simulink model "single_camera_xy_tracking_cv_ekf"  (R2025b)
settings: Solver=FixedStepDiscrete  StartTime=0  StopTime=T_end  FixedStep=Ts  RelTol=1e-3
InitFcn:
  | config_dir=fullfile(fileparts(get_param(bdroot,'FileName')),'..','config');
  | addpath(config_dir);
  | init_single_camera_xy_tracking_cv_ekf;
values from neighbouring files (symbols this model uses):
  Kpx = parameters(3)    [build_single_camera_joint_velocity_direct.m]    (also in build_single_camera_joint_velocity_direct1.m)
  Kpy = parameters(4);",  "k_ff=parameters(5)    [build_single_camera_joint_velocity_direct.m]    (also in build_single_camera_joint_velocity_direct1.m)
  Z_hat = parameters(2)    [build_single_camera_joint_velocity_direct.m]    (also in build_single_camera_joint_velocity_direct1.m)
undefined symbols (not defined in the file or in its folder): a_xy_max, command_velocity_timeout_sec, controller_enable, cx, cy, data, data_SL_Info, ekf_gate_threshold, ekf_reset_timeout_sec, enable_ekf_feedforward, enable_proportional, ff_ramp_time, fx, fy, joint_state_timeout_sec, k_ff, measurement_reset_timeout, P0, Q_ekf, R_ekf, required_valid_frames, target_timeout_sec, Ts, v_xy_max
libraries: ros2lib x5, robotmaniplib x3
Description:
  | Camera-frame 4-state CV Kalman Filter with commanded camera motion input.
settings Model: Creator=ASUS  LastModifiedBy=ASUS
settings DataIOCC: SignalLogging=off

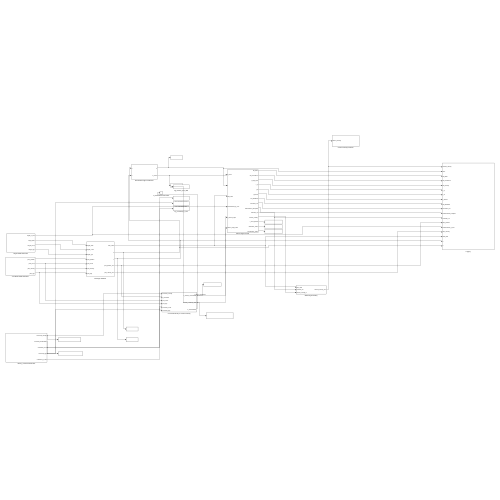
[thumbnail: Simulink's stored preview of the top-level diagram]
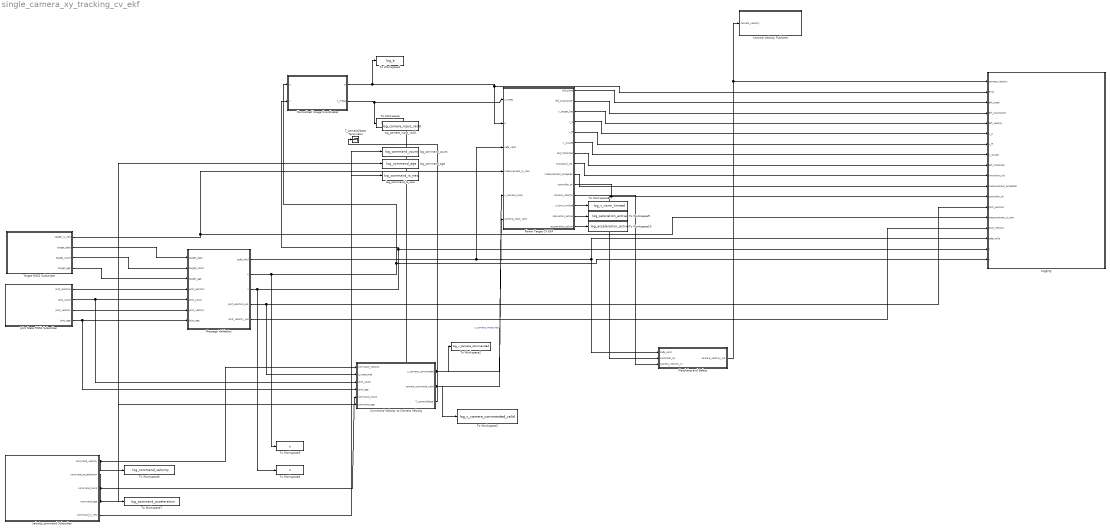
== system single_camera_xy_tracking_cv_ekf ==
  Camera Velocity Publisher : Subsystem
  Command Velocity to Camera Velocity : Subsystem
  Joint State ROS2 Subscriber : Subsystem
  Logging : Subsystem
  Message Validation : Subsystem
  Normalized Image Coordinates : Subsystem
  Planar Target CV EKF : Subsystem
  T_camera2base Terminator : Terminator
  Target ROS2 Subscriber : Subsystem
  To Workspace : ToWorkspace  VariableName=log_z_meas  SaveFormat=Timeseries  SampleTime=-1
  To Workspace1 : ToWorkspace  VariableName=log_e  SaveFormat=Timeseries  SampleTime=-1
  To Workspace10 : ToWorkspace  VariableName=log_acceleration_active  SaveFormat=Timeseries  SampleTime=-1
  To Workspace2 : ToWorkspace  VariableName=log_v_camera_commanded  SaveFormat=Timeseries  SampleTime=-1
  To Workspace3 : ToWorkspace  VariableName=log_v_camera_commanded_valid  SaveFormat=Timeseries  SampleTime=-1
  To Workspace4 : ToWorkspace  VariableName=v  SaveFormat=Timeseries  SampleTime=-1
  To Workspace5 : ToWorkspace  VariableName=u  SaveFormat=Timeseries  SampleTime=-1
  To Workspace6 : ToWorkspace  VariableName=log_command_velocity  SaveFormat=Timeseries  SampleTime=-1
  To Workspace7 : ToWorkspace  VariableName=log_command_acceleration  SaveFormat=Timeseries  SampleTime=-1
  To Workspace8 : ToWorkspace  VariableName=log_v_norm_limited  SaveFormat=Timeseries  SampleTime=-1
  To Workspace9 : ToWorkspace  VariableName=log_saturation_active  SaveFormat=Timeseries  SampleTime=-1
  Watchdog and Safety : Subsystem
  log_camera_input_valid : ToWorkspace  VariableName=log_camera_input_valid  SaveFormat=Timeseries  SampleTime=-1
  log_command_age : ToWorkspace  VariableName=log_command_age  SaveFormat=Timeseries  SampleTime=-1
  log_command_count : ToWorkspace  VariableName=log_command_count  SaveFormat=Timeseries  SampleTime=-1
  log_command_is_new : ToWorkspace  VariableName=log_command_is_new  SaveFormat=Timeseries  SampleTime=-1
  velocity_command Subscriber : Subsystem
  wires:
  Target ROS2 Subscriber/4(target_age) -> Message Validation/3(target_age)
  Target ROS2 Subscriber/2(target_data) -> Message Validation/1(target_data)
  Target ROS2 Subscriber/3(target_count) -> Message Validation/2(target_count)
  Planar Target CV EKF/3(v_target_hat) -> Logging/5(ekf_velocity)
  Message Validation/2(u) -> Normalized Image Coordinates/1(u), Logging/18(u), To Workspace5/1
  Planar Target CV EKF/10(controller_ok) -> Watchdog and Safety/2(controller_ok), Logging/12(controller_ok)
  Joint State ROS2 Subscriber/4(joint_age) -> Command Velocity to Camera Velocity/4(joint_age), Message Validation/7(joint_age)
  Joint State ROS2 Subscriber/2(joint_count) -> Command Velocity to Camera Velocity/3(joint_count), Message Validation/5(joint_count)
  Joint State ROS2 Subscriber/1(joint_position) -> Message Validation/4(joint_position)
  Joint State ROS2 Subscriber/3(joint_velocity) -> Message Validation/6(joint_velocity)
  Message Validation/1(safe_valid) -> Logging/16(safe_valid), Watchdog and Safety/1(safe_valid), Planar Target CV EKF/3(safe_valid)
  Message Validation/3(v) -> To Workspace4/1, Normalized Image Coordinates/2(v), Logging/17(v)
  Message Validation/4(joint_position_out) -> Command Velocity to Camera Velocity/2(q_measured), Logging/13(joint_position)
  Message Validation/5(joint_velocity_out) -> Logging/15(joint_velocity)
  Normalized Image Coordinates/1(e) -> To Workspace1/1, Logging/2(error), Planar Target CV EKF/2(e)
  Normalized Image Coordinates/2(z_meas) -> To Workspace/1, Planar Target CV EKF/1(z_meas)
  Planar Target CV EKF/1(ekf_state) -> Logging/3(ekf_state)
  Planar Target CV EKF/2(ekf_covariance) -> Logging/4(ekf_covariance)
  Planar Target CV EKF/9(measurement_accepted) -> Logging/11(measurement_accepted)
  Planar Target CV EKF/7(ekf_initialized) -> Logging/9(ekf_initialized)
  Planar Target CV EKF/8(innovation_nis) -> Logging/10(innovation_nis)
  Planar Target CV EKF/4(v_p) -> Logging/6(v_p)
  Planar Target CV EKF/5(v_ff) -> Logging/7(v_ff)
  Planar Target CV EKF/6(v_issued) -> Logging/8(v_issued)
  Planar Target CV EKF/11(camera_velocity) -> Watchdog and Safety/3(camera_velocity_in)
  Watchdog and Safety/1(camera_velocity_out) -> Camera Velocity Publisher/1(camera_velocity), Logging/1(camera_velocity)
  Target ROS2 Subscriber/1(target_is_new) -> Planar Target CV EKF/4(measurement_is_new), Logging/14(measurement_is_new)
  Command Velocity to Camera Velocity/1(v_camera_commanded) -> To Workspace2/1, Planar Target CV EKF/5(v_camera_input)  "v_camera_measured"
  Command Velocity to Camera Velocity/2(camera_command_valid) -> To Workspace3/1, Planar Target CV EKF/6(camera_input_valid), log_camera_input_valid/1
  velocity_command Subscriber/1(command_velocity) -> To Workspace6/1, Command Velocity to Camera Velocity/1(command_velocity)
  velocity_command Subscriber/2(command_acceleration) -> To Workspace7/1
  Planar Target CV EKF/12(v_norm_limited) -> To Workspace8/1
  Planar Target CV EKF/13(saturation_active) -> To Workspace9/1
  Planar Target CV EKF/14(acceleration_active) -> To Workspace10/1
  velocity_command Subscriber/3(command_count) -> Command Velocity to Camera Velocity/5(command_count), log_command_count/1
  velocity_command Subscriber/4(command_age) -> Command Velocity to Camera Velocity/6(command_age), log_command_age/1
  Command Velocity to Camera Velocity/3(T_camera2base) -> T_camera2base Terminator/1
  velocity_command Subscriber/5(command_is_new) -> log_command_is_new/1

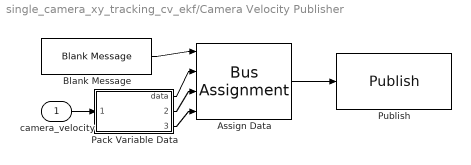
== system single_camera_xy_tracking_cv_ekf/Camera Velocity Publisher ==
  camera_velocity : Inport
  Assign Data : BusAssignment  AssignedSignals=data,data_SL_Info.CurrentLength,data_SL_Info.ReceivedLength
  Blank Message : ros2lib/Blank Message  messageClass=Message  entityType=std_msgs/Float64MultiArray  messageType=std_msgs/Float64MultiArray  SampleTime=Ts
  Pack Variable Data : MATLAB Function  TreatAsAtomicUnit=on
  Publish : ros2lib/Publish  topicSource=Select from ROS network  topic=/simulink/camera_velocity  messageType=std_msgs/Float64MultiArray  QOSHistory=Keep last  QOSDepth=1  QOSReliability=Reliable  QOSDurability=Volatile  QOSDeadline=Inf  QOSLifespan=Inf  QOSLiveliness=Automatic  QOSLeaseDuration=Inf  QOSAvoidROSNamespaceConventions=off
  wires:
  Blank Message/1 -> Assign Data/1
  Assign Data/1 -> Publish/1
  camera_velocity/1 -> Pack Variable Data/1(camera_velocity)
  Pack Variable Data/1(data) -> Assign Data/2
  Pack Variable Data/2(current_length) -> Assign Data/3
  Pack Variable Data/3(received_length) -> Assign Data/4

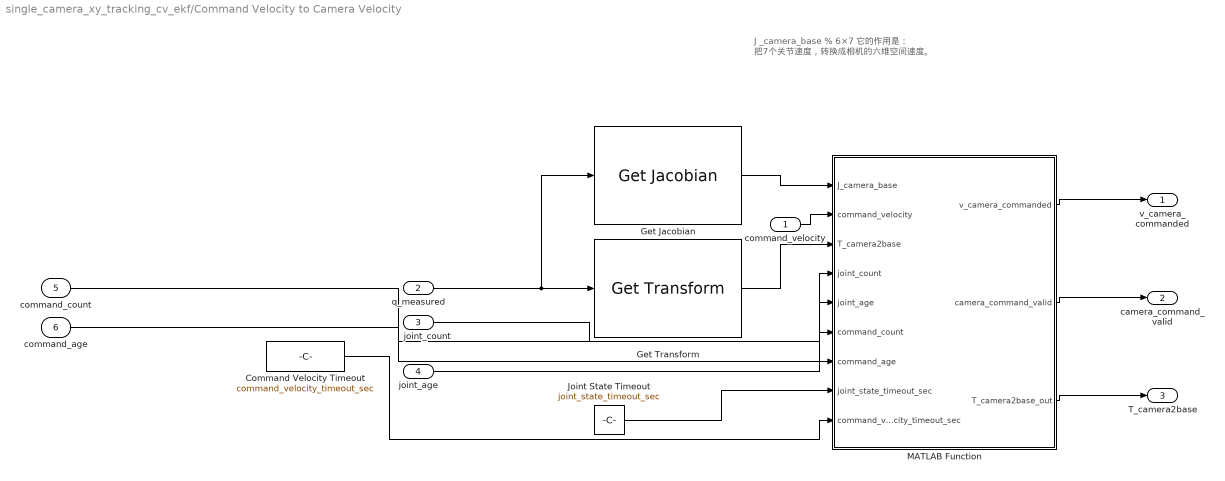
== system single_camera_xy_tracking_cv_ekf/Command Velocity to Camera Velocity ==
  note: J _camera_base % 6×7
      | 它的作用是：
      | 把7个关节速度，转换成相机的六维空间速度。
  command_velocity : Inport
  q_measured : Inport  Port=2
  joint_count : Inport  Port=3
  joint_age : Inport  Port=4
  command_count : Inport  Port=5
  command_age : Inport  Port=6
  Command Velocity Timeout : Constant  Value=command_velocity_timeout_sec
  Get Jacobian : robotmaniplib/Get Jacobian  RigidBodyTree=fr3_camera_robot  EndEffector=camera_link  SimulateUsing=Interpreted execution
  Get Transform : robotmaniplib/Get Transform  RigidBodyTree=fr3_camera_robot  SourceBody=camera_link  TargetBody=base  SimulateUsing=Interpreted execution
  Joint State Timeout : Constant  Value=joint_state_timeout_sec
  MATLAB Function : MATLAB Function  TreatAsAtomicUnit=on
  v_camera_commanded : Outport
  camera_command_valid : Outport  Port=2
  T_camera2base : Outport  Port=3
  wires:
  q_measured/1 -> Get Jacobian/1, Get Transform/1
  MATLAB Function/1(v_camera_commanded) -> v_camera_commanded/1
  MATLAB Function/2(camera_command_valid) -> camera_command_valid/1
  MATLAB Function/3(T_camera2base_out) -> T_camera2base/1
  Get Jacobian/1 -> MATLAB Function/1(J_camera_base)
  command_velocity/1 -> MATLAB Function/2(command_velocity)
  Get Transform/1 -> MATLAB Function/3(T_camera2base)
  joint_count/1 -> MATLAB Function/4(joint_count)
  joint_age/1 -> MATLAB Function/5(joint_age)
  command_count/1 -> MATLAB Function/6(command_count)
  command_age/1 -> MATLAB Function/7(command_age)
  Joint State Timeout/1 -> MATLAB Function/8(joint_state_timeout_sec)
  Command Velocity Timeout/1 -> MATLAB Function/9(command_velocity_timeout_sec)

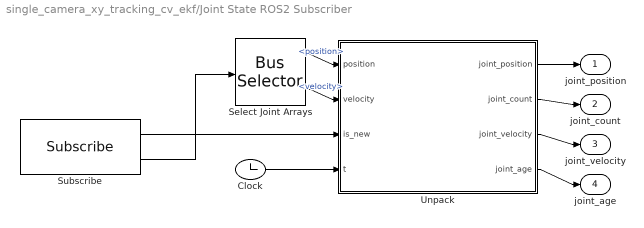
== system single_camera_xy_tracking_cv_ekf/Joint State ROS2 Subscriber ==
  Clock : Clock
  Select Joint Arrays : BusSelector  OutputSignals=position,velocity
  Subscribe : ros2lib/Subscribe  topicSource=Select from ROS network  topic=/franka/joint_states  messageType=sensor_msgs/JointState  sampleTime=Ts  QOSHistory=Keep last  QOSDepth=1  QOSReliability=Best effort  QOSDurability=Volatile  QOSDeadline=Inf  QOSLifespan=Inf  QOSLiveliness=Automatic  QOSLeaseDuration=Inf  QOSAvoidROSNamespaceConventions=off
  Unpack : MATLAB Function  TreatAsAtomicUnit=on
  joint_position : Outport
  joint_count : Outport  Port=2
  joint_velocity : Outport  Port=3
  joint_age : Outport  Port=4
  wires:
  Unpack/1(joint_position) -> joint_position/1
  Unpack/2(joint_count) -> joint_count/1
  Unpack/3(joint_velocity) -> joint_velocity/1
  Unpack/4(joint_age) -> joint_age/1
  Select Joint Arrays/1 -> Unpack/1(position)  "<position>"
  Select Joint Arrays/2 -> Unpack/2(velocity)  "<velocity>"
  Clock/1 -> Unpack/4(t)
  Subscribe/2 -> Select Joint Arrays/1
  Subscribe/1 -> Unpack/3(is_new)

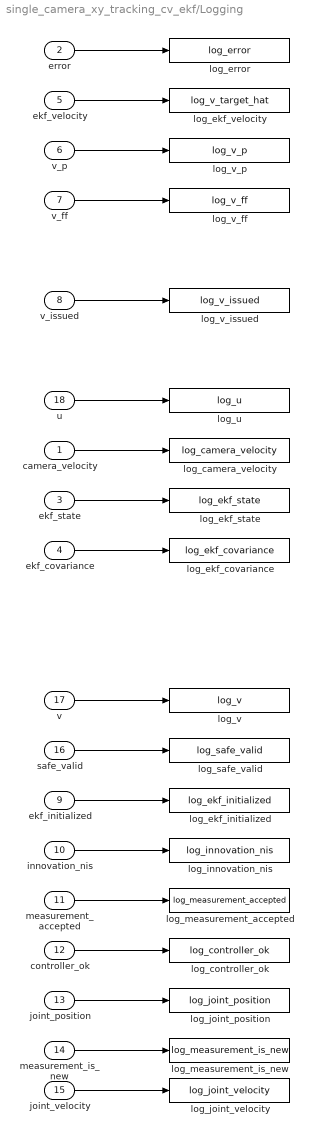
== system single_camera_xy_tracking_cv_ekf/Logging ==
  camera_velocity : Inport
  error : Inport  Port=2
  ekf_state : Inport  Port=3
  ekf_covariance : Inport  Port=4
  ekf_velocity : Inport  Port=5
  v_p : Inport  Port=6
  v_ff : Inport  Port=7
  v_issued : Inport  Port=8
  ekf_initialized : Inport  Port=9
  innovation_nis : Inport  Port=10
  measurement_accepted : Inport  Port=11
  controller_ok : Inport  Port=12
  joint_position : Inport  Port=13
  measurement_is_new : Inport  Port=14
  joint_velocity : Inport  Port=15
  safe_valid : Inport  Port=16
  v : Inport  Port=17
  u : Inport  Port=18
  log_camera_velocity : ToWorkspace  VariableName=log_camera_velocity  SaveFormat=Structure With Time  SampleTime=-1
  log_controller_ok : ToWorkspace  VariableName=log_controller_ok  SaveFormat=Structure With Time  SampleTime=-1
  log_ekf_covariance : ToWorkspace  VariableName=log_ekf_covariance  SaveFormat=Structure With Time  SampleTime=-1
  log_ekf_initialized : ToWorkspace  VariableName=log_ekf_initialized  SaveFormat=Structure With Time  SampleTime=-1
  log_ekf_state : ToWorkspace  VariableName=log_ekf_state  SaveFormat=Structure With Time  SampleTime=-1
  log_ekf_velocity : ToWorkspace  VariableName=log_v_target_hat  SaveFormat=Structure With Time  SampleTime=-1
  log_error : ToWorkspace  VariableName=log_error  SaveFormat=Structure With Time  SampleTime=-1
  log_innovation_nis : ToWorkspace  VariableName=log_innovation_nis  SaveFormat=Structure With Time  SampleTime=-1
  log_joint_position : ToWorkspace  VariableName=log_joint_position  SaveFormat=Structure With Time  SampleTime=-1
  log_joint_velocity : ToWorkspace  VariableName=log_joint_velocity  SaveFormat=Structure With Time  SampleTime=-1
  log_measurement_accepted : ToWorkspace  VariableName=log_measurement_accepted  SaveFormat=Structure With Time  SampleTime=-1
  log_measurement_is_new : ToWorkspace  VariableName=log_measurement_is_new  SaveFormat=Structure With Time  SampleTime=-1
  log_safe_valid : ToWorkspace  VariableName=log_safe_valid  SaveFormat=Structure With Time  SampleTime=-1
  log_u : ToWorkspace  VariableName=log_u  SaveFormat=Structure With Time  SampleTime=-1
  log_v : ToWorkspace  VariableName=log_v  SaveFormat=Structure With Time  SampleTime=-1
  log_v_ff : ToWorkspace  VariableName=log_v_ff  SaveFormat=Structure With Time  SampleTime=-1
  log_v_issued : ToWorkspace  VariableName=log_v_issued  SaveFormat=Structure With Time  SampleTime=-1
  log_v_p : ToWorkspace  VariableName=log_v_p  SaveFormat=Structure With Time  SampleTime=-1
  wires:
  error/1 -> log_error/1
  ekf_velocity/1 -> log_ekf_velocity/1
  v_p/1 -> log_v_p/1
  v_ff/1 -> log_v_ff/1
  v_issued/1 -> log_v_issued/1
  u/1 -> log_u/1
  camera_velocity/1 -> log_camera_velocity/1
  ekf_state/1 -> log_ekf_state/1
  ekf_covariance/1 -> log_ekf_covariance/1
  v/1 -> log_v/1
  safe_valid/1 -> log_safe_valid/1
  ekf_initialized/1 -> log_ekf_initialized/1
  innovation_nis/1 -> log_innovation_nis/1
  measurement_accepted/1 -> log_measurement_accepted/1
  controller_ok/1 -> log_controller_ok/1
  joint_position/1 -> log_joint_position/1
  joint_velocity/1 -> log_joint_velocity/1
  measurement_is_new/1 -> log_measurement_is_new/1

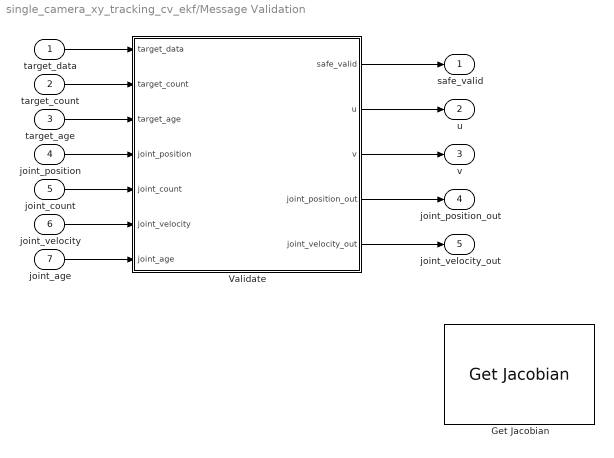
== system single_camera_xy_tracking_cv_ekf/Message Validation ==
  target_data : Inport
  target_count : Inport  Port=2
  target_age : Inport  Port=3
  joint_position : Inport  Port=4
  joint_count : Inport  Port=5
  joint_velocity : Inport  Port=6
  joint_age : Inport  Port=7
  Get Jacobian : robotmaniplib/Get Jacobian  RigidBodyTree=twoJointRigidBodyTree  EndEffector=tool  SimulateUsing=Interpreted execution
  Validate : MATLAB Function  TreatAsAtomicUnit=on
  safe_valid : Outport
  u : Outport  Port=2
  v : Outport  Port=3
  joint_position_out : Outport  Port=4
  joint_velocity_out : Outport  Port=5
  wires:
  Validate/1(safe_valid) -> safe_valid/1
  Validate/2(u) -> u/1
  Validate/3(v) -> v/1
  Validate/4(joint_position_out) -> joint_position_out/1
  Validate/5(joint_velocity_out) -> joint_velocity_out/1
  target_data/1 -> Validate/1(target_data)
  target_count/1 -> Validate/2(target_count)
  target_age/1 -> Validate/3(target_age)
  joint_position/1 -> Validate/4(joint_position)
  joint_count/1 -> Validate/5(joint_count)
  joint_velocity/1 -> Validate/6(joint_velocity)
  joint_age/1 -> Validate/7(joint_age)

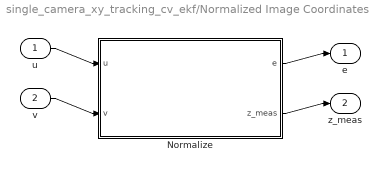
== system single_camera_xy_tracking_cv_ekf/Normalized Image Coordinates ==
  u : Inport
  v : Inport  Port=2
  Normalize : MATLAB Function  TreatAsAtomicUnit=on
  e : Outport
  z_meas : Outport  Port=2
  wires:
  u/1 -> Normalize/1(u)
  v/1 -> Normalize/2(v)
  Normalize/1(e) -> e/1
  Normalize/2(z_meas) -> z_meas/1

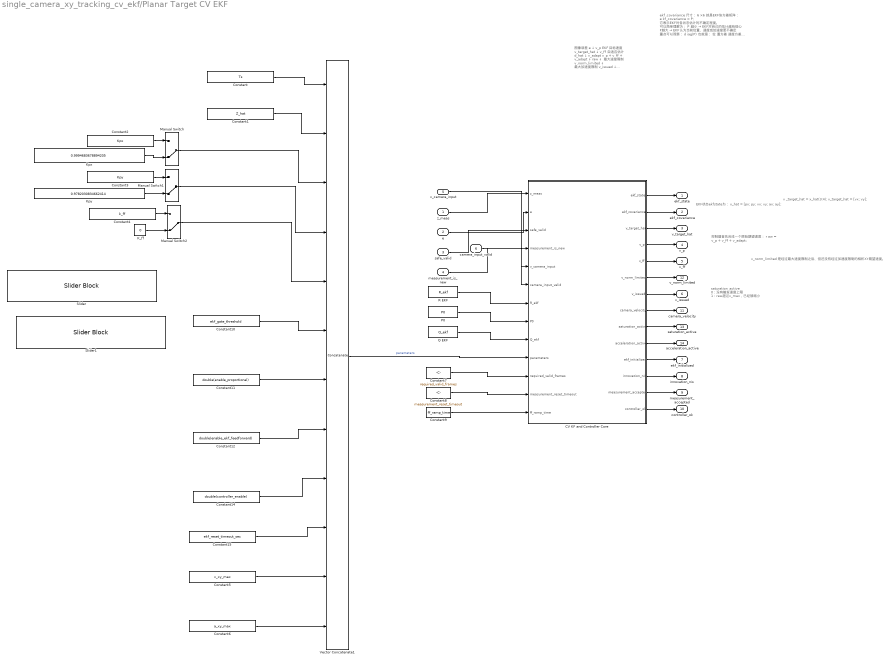
== system single_camera_xy_tracking_cv_ekf/Planar Target CV EKF ==
  note: saturation_active
      | 0：没有触发速度上限
      | 1：raw超过v_max，已经被缩小
  note: ekf_covariance
      | 尺寸：
      | 6 ×6
      | 就是EKF协方差矩阵：
      | e kf_covariance = P;
      | 它表示EKF对各状态估计的不确定程度。
      | 可以简单理解为：
      | P 越小
      | → EKF对自己的估计越有信心
      |
      | P越大
      | → EKF认为当前位置、速度或加速度更不确定
      | 重点可以观察：
      | d iag(P)
      | 也就是：
      | 位 置方差
      | 速度方差
      | 加速度方差
  note: 图像误差 e
      |     ↓
      | v_p
      |
      | EKF目标速度 v_target_hat
      |     ↓
      | v_ff
      |
      | 自适应估计 d_hat
      |     ↓
      | v_adapt
      |
      | v_p + v_ff + v_adapt
      |     ↓
      | raw
      |     ↓ 最大速度限制
      | v_norm_limited
      |     ↓ 最大加速度限制
      | v_issued
      |     ↓ 扩展为6维
      | camera_velocity
  note: EKF状态ekfstate为： x_hat = [px; py; vx; vy; ax; ay];
  note: v _target_hat = x_hat(3:4); v_target_hat = [vx; vy];
  note: 控制器首先合成一个原始期望速度：
      | r aw = v_p + v_ff + v_adapt;
  note: v_norm_limited 是经过最大速度限制之后、但还没有经过加速度限制的相机XY期望速度。
  z_meas : Inport
  e : Inport  Port=2
  safe_valid : Inport  Port=3
  measurement_is_new : Inport  Port=4
  v_camera_input : Inport  Port=5
  camera_input_valid : Inport  Port=6
  CV KF and Controller Core : MATLAB Function  TreatAsAtomicUnit=on
  Constant : Constant  Value=Ts
  Constant1 : Constant  Value=Z_hat
  Constant10 : Constant  Value=ekf_gate_threshold
  Constant11 : Constant  Value=double(enable_proportional)
  Constant12 : Constant  Value=double(enable_ekf_feedforward)
  Constant14 : Constant  Value=double(controller_enable)
  Constant15 : Constant  Value=ekf_reset_timeout_sec
  Constant2 : Constant  Value=Kpx
  Constant3 : Constant  Value=Kpy
  Constant4 : Constant  Value=k_ff
  Constant5 : Constant  Value=v_xy_max
  Constant6 : Constant  Value=a_xy_max
  Constant7 : Constant  Value=required_valid_frames
  Constant8 : Constant  Value=measurement_reset_timeout
  Constant9 : Constant  Value=ff_ramp_time
  K_ff : Constant  Value=0
  Kpx : Constant  Value=0.9994683678894205
  Kpy : Constant  Value=0.9782030834662414
  Manual Switch : ManualSwitch  CurrentSetting=0
  Manual Switch1 : ManualSwitch  CurrentSetting=0
  Manual Switch2 : ManualSwitch  CurrentSetting=0
  P0 : Constant  Value=P0
  Q EKF : Constant  Value=Q_ekf
  R EKF : Constant  Value=R_ekf
  Slider : SliderBlock  ScaleMax=10
  Slider1 : SliderBlock  ScaleMax=10
  Vector Concatenate1 : Concatenate  NumInputs=12
  ekf_state : Outport
  ekf_covariance : Outport  Port=2
  v_target_hat : Outport  Port=3
  v_p : Outport  Port=4
  v_ff : Outport  Port=5
  v_issued : Outport  Port=6
  ekf_initialized : Outport  Port=7
  innovation_nis : Outport  Port=8
  measurement_accepted : Outport  Port=9
  controller_ok : Outport  Port=10
  camera_velocity : Outport  Port=11
  v_norm_limited : Outport  Port=12
  saturation_active : Outport  Port=13
  acceleration_active : Outport  Port=14
  wires:
  CV KF and Controller Core/1(ekf_state) -> ekf_state/1
  CV KF and Controller Core/2(ekf_covariance) -> ekf_covariance/1
  CV KF and Controller Core/3(v_target_hat) -> v_target_hat/1
  CV KF and Controller Core/4(v_p) -> v_p/1
  CV KF and Controller Core/5(v_ff) -> v_ff/1
  CV KF and Controller Core/7(v_issued) -> v_issued/1
  CV KF and Controller Core/8(camera_velocity) -> camera_velocity/1
  CV KF and Controller Core/11(ekf_initialized) -> ekf_initialized/1
  CV KF and Controller Core/12(innovation_nis) -> innovation_nis/1
  CV KF and Controller Core/13(measurement_accepted) -> measurement_accepted/1
  CV KF and Controller Core/14(controller_ok) -> controller_ok/1
  Constant/1 -> Vector Concatenate1/1
  Constant1/1 -> Vector Concatenate1/2
  Constant10/1 -> Vector Concatenate1/6
  Constant11/1 -> Vector Concatenate1/7
  Constant12/1 -> Vector Concatenate1/8
  Constant14/1 -> Vector Concatenate1/9
  Constant15/1 -> Vector Concatenate1/10
  Constant2/1 -> Manual Switch/1
  Manual Switch/1 -> Vector Concatenate1/3
  Kpx/1 -> Manual Switch/2
  Kpy/1 -> Manual Switch1/2
  Constant3/1 -> Manual Switch1/1
  Manual Switch1/1 -> Vector Concatenate1/4
  Constant4/1 -> Manual Switch2/1
  Manual Switch2/1 -> Vector Concatenate1/5
  K_ff/1 -> Manual Switch2/2
  CV KF and Controller Core/6(v_norm_limited) -> v_norm_limited/1
  CV KF and Controller Core/10(acceleration_active) -> acceleration_active/1
  CV KF and Controller Core/9(saturation_active) -> saturation_active/1
  Constant6/1 -> Vector Concatenate1/12
  Constant5/1 -> Vector Concatenate1/11
  z_meas/1 -> CV KF and Controller Core/1(z_meas)
  e/1 -> CV KF and Controller Core/2(e)
  safe_valid/1 -> CV KF and Controller Core/3(safe_valid)
  measurement_is_new/1 -> CV KF and Controller Core/4(measurement_is_new)
  v_camera_input/1 -> CV KF and Controller Core/5(v_camera_input)
  camera_input_valid/1 -> CV KF and Controller Core/6(camera_input_valid)
  R EKF/1 -> CV KF and Controller Core/7(R_ekf)
  P0/1 -> CV KF and Controller Core/8(P0)
  Q EKF/1 -> CV KF and Controller Core/9(Q_ekf)
  Vector Concatenate1/1 -> CV KF and Controller Core/10(parameters)  "parameters"
  Constant7/1 -> CV KF and Controller Core/11(required_valid_frames)
  Constant8/1 -> CV KF and Controller Core/12(measurement_reset_timeout)
  Constant9/1 -> CV KF and Controller Core/13(ff_ramp_time)

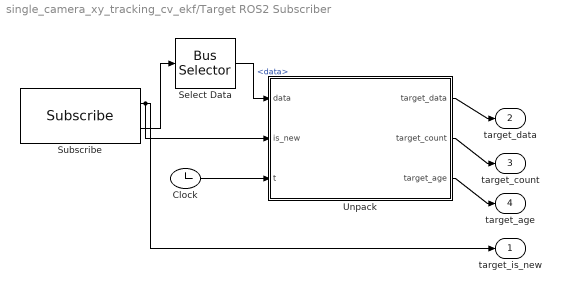
== system single_camera_xy_tracking_cv_ekf/Target ROS2 Subscriber ==
  Clock : Clock
  Select Data : BusSelector  OutputSignals=data
  Subscribe : ros2lib/Subscribe  topicSource=Select from ROS network  topic=/apriltag_detector/target_position  messageType=std_msgs/Float64MultiArray  sampleTime=Ts  QOSHistory=Keep last  QOSDepth=1  QOSReliability=Best effort  QOSDurability=Volatile  QOSDeadline=Inf  QOSLifespan=Inf  QOSLiveliness=Automatic  QOSLeaseDuration=Inf  QOSAvoidROSNamespaceConventions=off
  Unpack : MATLAB Function  TreatAsAtomicUnit=on
  target_is_new : Outport
  target_data : Outport  Port=2
  target_count : Outport  Port=3
  target_age : Outport  Port=4
  wires:
  Unpack/1(target_data) -> target_data/1
  Unpack/2(target_count) -> target_count/1
  Unpack/3(target_age) -> target_age/1
  Select Data/1 -> Unpack/1(data)  "<data>"
  Clock/1 -> Unpack/3(t)
  Subscribe/2 -> Select Data/1
  Subscribe/1 -> Unpack/2(is_new), target_is_new/1

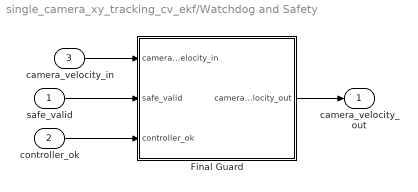
== system single_camera_xy_tracking_cv_ekf/Watchdog and Safety ==
  safe_valid : Inport
  controller_ok : Inport  Port=2
  camera_velocity_in : Inport  Port=3
  Final Guard : MATLAB Function  TreatAsAtomicUnit=on
  camera_velocity_out : Outport
  wires:
  camera_velocity_in/1 -> Final Guard/1(camera_velocity_in)
  safe_valid/1 -> Final Guard/2(safe_valid)
  controller_ok/1 -> Final Guard/3(controller_ok)
  Final Guard/1(camera_velocity_out) -> camera_velocity_out/1

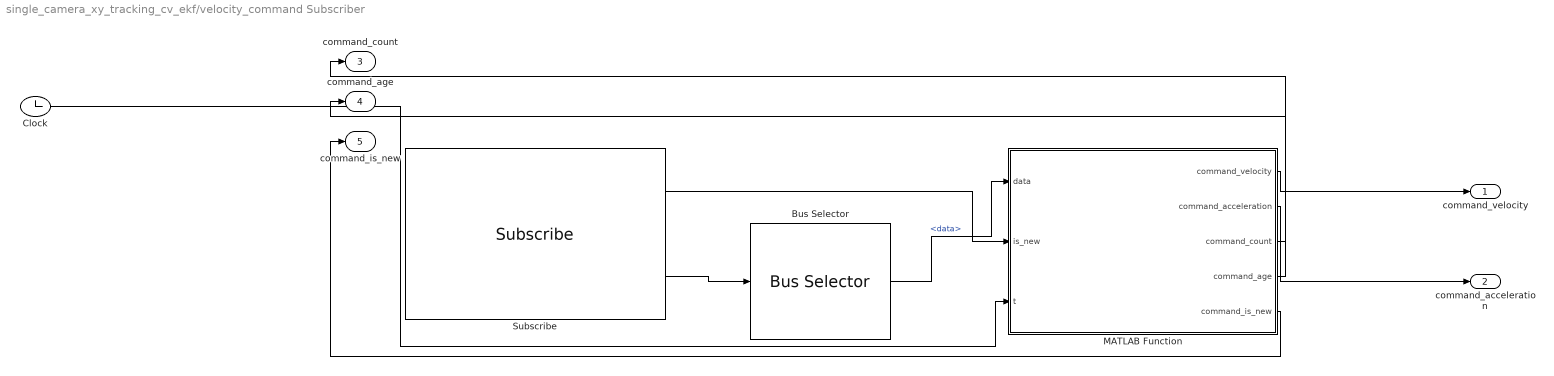
== system single_camera_xy_tracking_cv_ekf/velocity_command Subscriber ==
  Bus Selector : BusSelector  OutputSignals=data
  Clock : Clock
  MATLAB Function : MATLAB Function  TreatAsAtomicUnit=on
  Subscribe : ros2lib/Subscribe  topicSource=Specify your own  topic=/joint_velocity_example_controller/commands  messageType=std_msgs/Float64MultiArray  sampleTime=-1  QOSHistory=Keep last  QOSDepth=10  QOSReliability=Reliable  QOSDurability=Volatile  QOSDeadline=Inf  QOSLifespan=Inf  QOSLiveliness=Automatic  QOSLeaseDuration=Inf  QOSAvoidROSNamespaceConventions=off
  command_velocity : Outport
  command_acceleration : Outport  Port=2
  command_count : Outport  Port=3
  command_age : Outport  Port=4
  command_is_new : Outport  Port=5
  wires:
  Subscribe/2 -> Bus Selector/1
  Bus Selector/1 -> MATLAB Function/1(data)  "<data>"
  MATLAB Function/2(command_acceleration) -> command_acceleration/1
  MATLAB Function/1(command_velocity) -> command_velocity/1
  Subscribe/1 -> MATLAB Function/2(is_new)
  Clock/1 -> MATLAB Function/3(t)
  MATLAB Function/3(command_count) -> command_count/1
  MATLAB Function/4(command_age) -> command_age/1
  MATLAB Function/5(command_is_new) -> command_is_new/1

== matlab function single_camera_xy_tracking_cv_ekf/Planar Target CV EKF/CV KF and Controller Core ==
  data: z_meas input size=[2 1]; e input size=[2 1]; safe_valid input size=1; measurement_is_new input size=1; v_camera_input input size=[2 1]; camera_input_valid input size=1; ekf_state output size=[4 1]; R_ekf input size=[2 2]; P0 input size=[4 4]; Q_ekf input size=[4 4]; parameters input size=[12 1]; ekf_covariance output size=[4 4]; v_target_hat output size=[2 1]; v_p output size=[2 1]; v_ff output size=[2 1]; v_norm_limited output size=[2 1]; v_issued output size=[2 1]; camera_velocity output size=[6 1]; saturation_active output; acceleration_active output; ekf_initialized output size=1; innovation_nis output size=1; measurement_accepted output size=1; controller_ok output size=1; required_valid_frames input size=1; measurement_reset_timeout input size=1; ff_ramp_time input size=1
function [ekf_state,ekf_covariance,v_target_hat,v_p,v_ff, ...
    v_norm_limited,v_issued,camera_velocity,saturation_active, ...
    acceleration_active,ekf_initialized,innovation_nis, ...
    measurement_accepted,controller_ok]=fcn( ...
    z_meas,e,safe_valid,measurement_is_new,v_camera_input, ...
    camera_input_valid,R_ekf,P0,Q_ekf,parameters, ...
    required_valid_frames,measurement_reset_timeout,ff_ramp_time)
%#codegen
% 带相机运动输入的四状态匀速滤波器及P+速度前馈控制器。
% 状态：[X_C;Y_C;V_tx,C;V_ty,C]，测量和速度均在相机坐标系表达。
% 适用条件：固定Z_hat、相机仅XY平移、vz=0、角速度=0、忽略姿态变化。
% 系统和测量方程均为线性；保留EKF名称仅为兼容现有项目结构。
persistent x P e_hold elapsed initialized v_previous valid_streak ekf_ready ff_ramp
if isempty(initialized)
    x=zeros(4,1); P=P0; e_hold=zeros(2,1); elapsed=0;
    initialized=false; v_previous=zeros(2,1); valid_streak=0;
    ekf_ready=false; ff_ramp=0;
end

ekf_state=x; ekf_covariance=P; v_target_hat=zeros(2,1);
v_p=zeros(2,1); v_ff=zeros(2,1); v_norm_limited=zeros(2,1);
v_issued=zeros(2,1); camera_velocity=zeros(6,1);
saturation_active=false; acceleration_active=false;
ekf_initialized=initialized&&ekf_ready; innovation_nis=NaN;
measurement_accepted=false; controller_ok=false;

if numel(parameters)<12, x(:)=0; P=P0; initialized=false; ekf_ready=false; return; end
Ts=parameters(1); Z_hat=parameters(2); Kp=parameters(3:4);
k_ff=parameters(5); gate=parameters(6); enable_p=parameters(7)>.5;
enable_ff=parameters(8)>.5; controller_enable=parameters(9)>.5;
v_xy_max=parameters(11); a_xy_max=parameters(12);
safe_valid=safe_valid>.5; measurement_is_new=measurement_is_new>.5;
required_valid_frames=max(1,floor(required_valid_frames));
parameter_ok=all(isfinite(parameters(:))) && ...
    isfinite(required_valid_frames) && isfinite(measurement_reset_timeout) && ...
    isfinite(ff_ramp_time) && Ts>0 && Z_hat>0 && gate>0 && ...
    measurement_reset_timeout>=Ts && ff_ramp_time>0 && ...
    v_xy_max>0 && a_xy_max>0 && isequal(size(P0),[4 4]) && ...
    isequal(size(Q_ekf),[4 4]) && isequal(size(R_ekf),[2 2]) && ...
    all(isfinite(P0(:))) && all(isfinite(Q_ekf(:))) && all(isfinite(R_ekf(:)));
if ~parameter_ok
    x(:)=0; P=P0; e_hold(:)=0; elapsed=0; initialized=false;
    v_previous(:)=0; valid_streak=0; ekf_ready=false; ff_ramp=0;
    ekf_state=x; ekf_covariance=P; ekf_initialized=false; return
end

A=[1 0 Ts 0;0 1 0 Ts;0 0 1 0;0 0 0 1];
B=[-Ts 0;0 -Ts;0 0;0 0];
H=[1 0 0 0;0 1 0 0];
vectors_ok=numel(z_meas)==2 && numel(e)==2 && ...
    all(isfinite(z_meas(:))) && all(isfinite(e(:)));
current_visual_valid=safe_valid&&vectors_ok;
measurement_available=current_visual_valid&&measurement_is_new;
z_camera=zeros(2,1);
if vectors_ok, z_camera=reshape(z_meas,2,1); end

input_ok=camera_input_valid>.5 && numel(v_camera_input)==2 && ...
    all(isfinite(v_camera_input(:)));
u_used=zeros(2,1);
if input_ok, u_used=reshape(v_camera_input,2,1); end

if ~initialized
    if measurement_available
        x=[z_camera;0;0]; P=P0; initialized=true; measurement_accepted=true;
    end
else
    [x,P,innovation_nis,measurement_accepted]=cv_ekf_step( ...
        x,P,z_camera,u_used,measurement_available,A,B,H,Q_ekf,R_ekf,gate);
end

if current_visual_valid&&measurement_is_new, e_hold=reshape(e,2,1); end
if measurement_accepted
    elapsed=0; valid_streak=min(valid_streak+1,required_valid_frames);
    if valid_streak>=required_valid_frames, ekf_ready=true; end
else
    if measurement_is_new&&~ekf_ready, valid_streak=0; end
    elapsed=elapsed+Ts;
end

state_ok=all(isfinite(x)) && all(isfinite(P(:))) && ...
    all(diag(P)>=0) && norm(P-P','fro')<1e-6;
if elapsed>=measurement_reset_timeout || ~state_ok
    x(:)=0; P=P0; e_hold(:)=0; elapsed=0; initialized=false;
    v_previous(:)=0; valid_streak=0; ekf_ready=false; ff_ramp=0;
    ekf_state=x; ekf_covariance=P; ekf_initialized=false; return
end

if ~current_visual_valid
    e_hold(:)=0; v_previous(:)=0; ff_ramp=0;
    ekf_state=x; ekf_covariance=P;
    if ekf_ready, v_target_hat=x(3:4); else, ekf_state(3:4)=0; end
    ekf_initialized=initialized&&ekf_ready; return
end

ekf_state=x; ekf_covariance=P;
if ekf_ready, v_target_hat=x(3:4); else, ekf_state(3:4)=0; end
ekf_initialized=initialized&&ekf_ready;
if ~controller_enable||~initialized
    v_previous(:)=0; ff_ramp=0; return
end

if enable_p, v_p=Z_hat*Kp.*e_hold; end
if enable_ff&&ekf_ready
    ff_ramp=min(1,ff_ramp+Ts/ff_ramp_time);
    v_ff=ff_ramp*k_ff*x(3:4);
else
    ff_ramp=0;
end
raw=v_p+v_ff; raw_norm=norm(raw); saturation_active=raw_norm>v_xy_max;
if saturation_active, v_norm_limited=raw*(v_xy_max/raw_norm); else, v_norm_limited=raw; end
delta=v_norm_limited-v_previous; delta_norm=norm(delta); delta_max=a_xy_max*Ts;
acceleration_active=delta_norm>delta_max;
if acceleration_active
    v_issued=v_previous+delta*(delta_max/delta_norm);
else
    v_issued=v_norm_limited;
end
controller_ok=all(isfinite([v_p;v_ff;v_norm_limited;v_issued]));
if controller_ok
    v_previous=v_issued;
    camera_velocity=[v_issued;0;0;0;0];
else
    v_p(:)=0; v_ff(:)=0; v_norm_limited(:)=0; v_issued(:)=0;
    saturation_active=false; acceleration_active=false;
    v_previous(:)=0; ff_ramp=0; camera_velocity(:)=0;
end
end

== matlab function single_camera_xy_tracking_cv_ekf/Watchdog and Safety/Final Guard ==
  data: camera_velocity_in input size=[6 1]; camera_velocity_out output size=[6 1]; safe_valid input size=1; controller_ok input size=1
function camera_velocity_out = fcn(camera_velocity_in,safe_valid,controller_ok)
%#codegen
camera_velocity_out=zeros(6,1);
if safe_valid && controller_ok && all(isfinite(camera_velocity_in(:)))
    camera_velocity_out=camera_velocity_in;
    camera_velocity_out(3:6)=0;
end
end

== matlab function single_camera_xy_tracking_cv_ekf/Camera Velocity Publisher/Pack Variable Data ==
  data: camera_velocity input size=[6 1]; data output size=[128 1]; current_length output size=1; received_length output size=1
function [data,current_length,received_length] = fcn(camera_velocity)
%#codegen
data=zeros(128,1); data(1:6)=camera_velocity;
current_length=uint32(6); received_length=uint32(6);
end

== matlab function single_camera_xy_tracking_cv_ekf/velocity_command Subscriber/MATLAB Function ==
  data: data input; is_new input size=1; command_velocity output size=[7 1]; command_acceleration output size=[7 1]; t input size=1; command_count output size=1; command_age output size=1; command_is_new output size=1
function [command_velocity,command_acceleration,command_count, ...
    command_age,command_is_new]=fcn(data,is_new,t)
%#codegen
% 缓存最近一次合法的7关节命令速度，并输出消息年龄和新鲜度。
persistent last_velocity last_time last_count previous_velocity initialized
if isempty(initialized)
    last_velocity=zeros(7,1); previous_velocity=zeros(7,1);
    last_time=-1e6; last_count=0; initialized=false;
end
command_velocity=last_velocity; command_acceleration=zeros(7,1);
command_count=last_count; command_age=max(0,t-last_time);
command_is_new=false;
if ~is_new || numel(data)<7, return; end

current=zeros(7,1); valid=true;
for k=1:7
    current(k)=double(data(k)); valid=valid&&isfinite(current(k));
end
if ~valid, return; end
if initialized, command_acceleration=(current-previous_velocity)*120; end
last_velocity=current; previous_velocity=current; last_time=t;
last_count=7; initialized=true;
command_velocity=current; command_count=7; command_age=0;
command_is_new=true;
end

== matlab function single_camera_xy_tracking_cv_ekf/Target ROS2 Subscriber/Unpack ==
  data: data input; target_data output size=[3 1]; is_new input size=1; t input size=1; target_count output size=1; target_age output size=1
function [target_data,target_count,target_age] = fcn(data,is_new,t)
%#codegen
persistent last_data last_count last_time
if isempty(last_count), last_data=zeros(3,1); last_count=0.0; last_time=-1.0e6; end
if is_new
    n=numel(data); last_data=zeros(3,1);
    if n>=1, last_data(1)=data(1); end
    if n>=2, last_data(2)=data(2); end
    if n>=3, last_data(3)=data(3); end
    last_count=double(n); last_time=t;
end
target_data=last_data; target_count=last_count; target_age=max(0.0,t-last_time);
end

== matlab function single_camera_xy_tracking_cv_ekf/Command Velocity to Camera Velocity/MATLAB Function ==
  data: J_camera_base input size=[6 7]; v_camera_commanded output size=[2 1]; command_velocity input size=[7 1]; T_camera2base input size=[4 4]; joint_count input size=1; joint_age input size=1; command_count input size=1; camera_command_valid output size=1; T_camera2base_out output size=[4 4]; command_age input size=1; joint_state_timeout_sec input size=1; command_velocity_timeout_sec input size=1
function [v_camera_commanded,camera_command_valid,T_camera2base_out]=fcn( ...
    J_camera_base,command_velocity,T_camera2base,joint_count,joint_age, ...
    command_count,command_age,joint_state_timeout_sec, ...
    command_velocity_timeout_sec)
%#codegen
% 用当前关节位置的雅可比把最终关节命令换算为相机系XY线速度。
[v_camera_commanded,camera_command_valid]=command_to_camera_velocity( ...
    J_camera_base,command_velocity,T_camera2base,joint_count,joint_age, ...
    command_count,command_age,joint_state_timeout_sec, ...
    command_velocity_timeout_sec);
T_camera2base_out=T_camera2base;
end

== matlab function single_camera_xy_tracking_cv_ekf/Joint State ROS2 Subscriber/Unpack ==
  data: position input; joint_position output size=[7 1]; velocity input; is_new input size=1; t input size=1; joint_count output size=1; joint_velocity output size=[7 1]; joint_age output size=1
function [joint_position,joint_count,joint_velocity,joint_age] = fcn(position,velocity,is_new,t)
%#codegen
persistent last_q last_dq last_count last_time
if isempty(last_count), last_q=zeros(7,1); last_dq=zeros(7,1); last_count=0.0; last_time=-1.0e6; end
if is_new
    np=numel(position); nv=numel(velocity); last_q=zeros(7,1); last_dq=zeros(7,1);
    for k=1:min(np,7), last_q(k)=position(k); end
    for k=1:min(nv,7), last_dq(k)=velocity(k); end
    last_count=double(min(np,nv)); last_time=t;
end
joint_position=last_q; joint_count=last_count; joint_velocity=last_dq; joint_age=max(0.0,t-last_time);
end

== matlab function single_camera_xy_tracking_cv_ekf/Message Validation/Validate ==
  data: target_data input size=[3 1]; safe_valid output size=1; target_count input size=1; target_age input size=1; joint_position input size=[7 1]; joint_count input size=1; joint_velocity input size=[7 1]; joint_age input size=1; u output size=1; v output size=1; joint_position_out output size=[7 1]; joint_velocity_out output size=[7 1]; target_timeout_sec parameter size=1; joint_state_timeout_sec parameter size=1
function [safe_valid,u,v,joint_position_out,joint_velocity_out] = fcn(target_data,target_count,target_age,joint_position,joint_count,joint_velocity,joint_age, target_timeout_sec, joint_state_timeout_sec)
%#codegen
u=0.0; v=0.0; joint_position_out=zeros(7,1); joint_velocity_out=zeros(7,1);
target_ok=target_count>=3 && target_data(1)>0.5 && isfinite(target_data(2)) && isfinite(target_data(3)) && isfinite(target_age) && target_age<=target_timeout_sec;
joint_ok=joint_count>=7 && all(isfinite(joint_position(:))) && all(isfinite(joint_velocity(:))) && isfinite(joint_age) && joint_age<=joint_state_timeout_sec;
if target_ok, u=target_data(2); v=target_data(3); end
if joint_ok, joint_position_out=joint_position; joint_velocity_out=joint_velocity; end
safe_valid=target_ok && joint_ok;
end

== matlab function single_camera_xy_tracking_cv_ekf/Normalized Image Coordinates/Normalize ==
  data: u input size=1; e output size=[2 1]; v input size=1; z_meas output size=[2 1]; fx parameter size=1; fy parameter size=1; cx parameter size=1; cy parameter size=1; Z_hat parameter size=1
function [e,z_meas] = fcn(u,v, fx, fy, cx, cy, Z_hat)
%#codegen
ex=(u-cx)/fx; ey=(v-cy)/fy;
e=[ex;ey]; z_meas=Z_hat*e;
end
